simulink model "sailboatModel"  (R2017a)
settings: Solver=ode3  StartTime=0.0  StopTime=200  FixedStep=0.4  RelTol=1e-3
libraries: simulink x2
settings Model: Creator=Administrator  LastModifiedBy=davi
settings DataIOCC: LimitDataPoints=on  SaveFormat=Array  SignalLoggingSaveFormat=ModelDataLogs
settings OptimizationCC: BlockReduction=off  BooleanDataType=off  LifeSpan=inf
settings DebuggingCC: SaveWithParameterizedLinksMsg=none  UnderspecifiedInitializationDetection=Classic  MergeDetectMultiDrivingBlocksExec=none  SignalResolutionControl=TryResolveAllWithWarning  MultiTaskDSMMsg=warning  MultiTaskCondExecSysMsg=none  StateNameClashWarn=warning  SFUnexpectedBacktrackingDiag=warning  SFNoUnconditionalDefaultTransitionDiag=warning  SFExecutionAtInitializationDiag=none
settings HardwareCC: ProdBitPerPointer=32  ProdBitPerSizeT=32  ProdBitPerPtrDiffT=32  ProdLargestAtomicFloat=None  ProdIntDivRoundTo=Undefined  ProdEndianess=Unspecified  ProdWordSize=32  ProdHWDeviceType=32-bit Generic  TargetUnknown=on
settings ModelReferenceCC: PropagateSignalLabelsOutOfModel=off
settings GRTTargetCC: TargetLangStandard=C89/C90 (ANSI)  GeneratePreprocessorConditionals=Disable all
settings ConfigComp: CovMetricSettings=dw  CovHtmlReporting=on  CovSaveCumulativeToWorkspaceVar=on  CovSaveSingleToWorkspaceVar=on  CovExternalEMLEnable=off

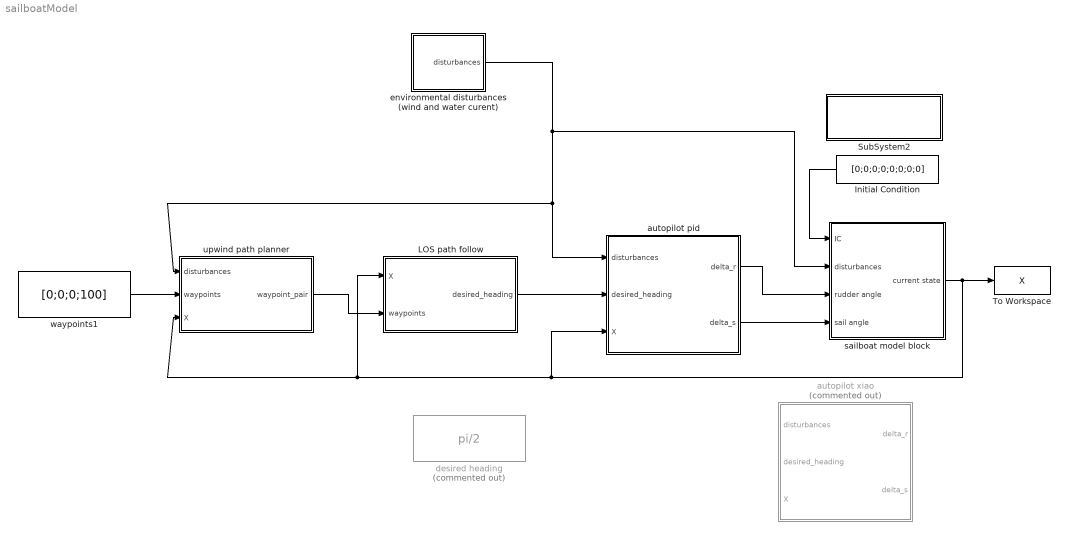
== system sailboatModel ==
  Initial Condition : Constant  Value=[0;0;0;0;0;0;0;0]
  LOS path follow : Subsystem
  SubSystem2 : Subsystem  InitFcn=init_par
      mask Display: disp('Parameter Initialization')
  To Workspace : ToWorkspace  VariableName=X  SaveFormat=Structure With Time  SampleTime=-1
  autopilot pid : Subsystem
  autopilot xiao : Subsystem  Commented=on
  desired heading : Constant  Commented=on  Value=pi/2
  environmental disturbances (wind and water curent) : Subsystem
  sailboat model block : Subsystem  StopFcn=|
      | %close all;
      | %plot(X.signals.values(:,1), X.signals.values(:,2),'r', 'LineWidth', 1.5);
      | %axis([-max(max(X.signals.values(:,1),max(X.signals.values(:,2))))/2 max(max(X.signals.values(:,1),max(X.signals.values(:,2))))/2 min(min(X.signals.values(:,1),min(X.signals.values(:,2)))) max(max(X.signals.values(:,1),max(X.signals.values(:,2))))]);
      | %grid;
      | %xlabel('x[m]');
      | %ylabel('y[m]');
      | %
      | %figure;
      | %hold on;
      | %plot(X.time, rad2deg(X.signals.values(:,4)),'r', 'LineWidth', 1.5);
      | %xlabel('Time[s]');
      | %ylabel('Heading[deg]');
      | %grid;
  upwind path planner : Subsystem
  waypoints1 : Constant  Value=[0;0;0;100]
  wires:
  sailboat model block/1(current state) -> autopilot pid/3(X), LOS path follow/1(X), upwind path planner/3(X), To Workspace/1
  Initial Condition/1 -> sailboat model block/1(IC)
  autopilot pid/1(delta_r) -> sailboat model block/3(rudder angle)
  autopilot pid/2(delta_s) -> sailboat model block/4(sail angle)
  environmental disturbances (wind and water curent)/1(disturbances) -> autopilot pid/1(disturbances), upwind path planner/1(disturbances), sailboat model block/2(disturbances)
  LOS path follow/1(desired_heading) -> autopilot pid/2(desired_heading)
  waypoints1/1 -> upwind path planner/2(waypoints)
  upwind path planner/1(waypoint_pair) -> LOS path follow/2(waypoints)

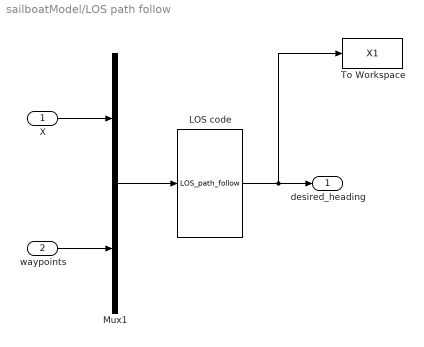
== system sailboatModel/LOS path follow ==
  X : Inport
  waypoints : Inport  Port=2
  LOS code : MATLABFcn  MATLABFcn=LOS_path_follow  OutputDimensions=1
  Mux1 : Mux  Inputs=2
  To Workspace : ToWorkspace  VariableName=X1  SaveFormat=Structure With Time  SampleTime=-1
  desired_heading : Outport
  wires:
  X/1 -> Mux1/1
  Mux1/1 -> LOS code/1
  LOS code/1 -> To Workspace/1, desired_heading/1
  waypoints/1 -> Mux1/2

== system sailboatModel/SubSystem2 ==

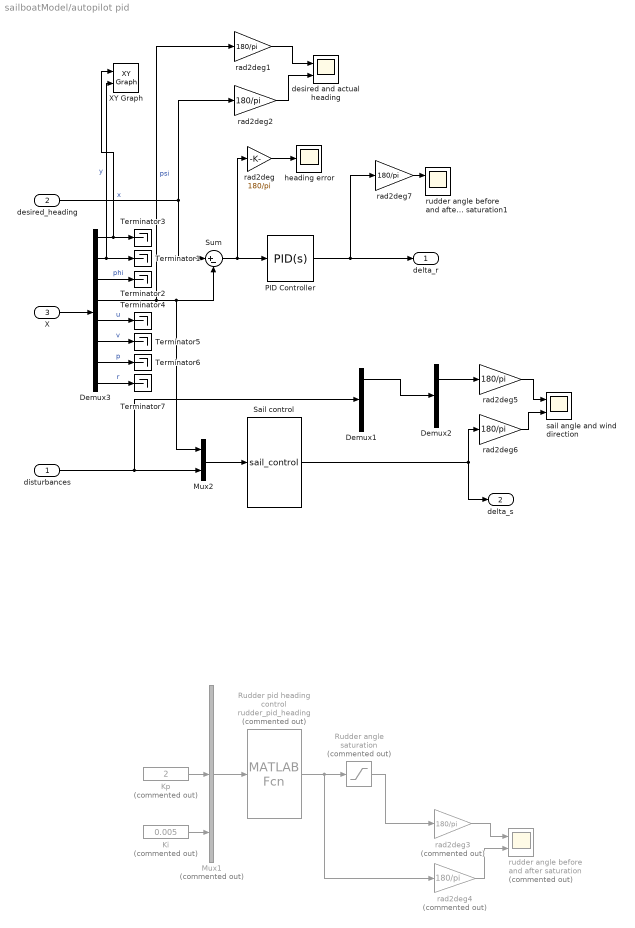
== system sailboatModel/autopilot pid ==
  disturbances : Inport
  desired_heading : Inport  Port=2
  X : Inport  Port=3
  Demux1 : Demux  Outputs=3
  Demux2 : Demux  Outputs=2
  Demux3 : Demux  Outputs=8
  Ki : Constant  Commented=on  Value=0.005
  Kp : Constant  Commented=on  Value=2
  Mux1 : Mux  Commented=on  Inputs=3
  Mux2 : Mux  Inputs=2
  PID Controller : simulink/Continuous/PID Controller  Controller=PID  TimeDomain=Continuous-time  SampleTime=-1  IntegratorMethod=Forward Euler  FilterMethod=Forward Euler  Form=Parallel  UseFilter=on  ControllerParametersSource=internal  P=3  I=0.05  D=0.5  N=1  InitialConditionSource=internal  InitialConditionForIntegrator=0  InitialConditionForFilter=0  ExternalReset=none  LimitOutput=on  UpperSaturationLimit=pi/3  LowerSaturationLimit=-pi/3  LinearizeAsGain=on  AntiWindupMode=clamping  Kb=1  TrackingMode=off  Kt=1  PParamMin=[]  PParamMax=[]  IParamMin=[]  IParamMax=[]  DParamMin=[]  DParamMax=[]  NParamMin=[]  NParamMax=[]  KbParamMin=[]  KbParamMax=[]  KtParamMin=[]  KtParamMax=[]  POutMin=[]  POutMax=[]  IOutMin=[]  IOutMax=[]  DOutMin=[]  DOutMax=[]  NOutMin=[]  NOutMax=[]  KbOutMin=[]  KbOutMax=[]  KtOutMin=[]  KtOutMax=[]  IntegratorOutMin=[]  IntegratorOutMax=[]  FilterOutMin=[]  FilterOutMax=[]  SumOutMin=[]  SumOutMax=[]  SumI1OutMin=[]  SumI1OutMax=[]  SumI2OutMin=[]  SumI2OutMax=[]  SumI3OutMin=[]  SumI3OutMax=[]  SumDOutMin=[]  SumDOutMax=[]  SaturationOutMin=[]  SaturationOutMax=[]  IntegratorContinuousStateAttributes=''  IntegratorStateMustResolveToSignalObject=off  IntegratorRTWStateStorageClass=Auto  FilterContinuousStateAttributes=''  FilterStateMustResolveToSignalObject=off  FilterRTWStateStorageClass=Auto  DifferentiatorICPrevScaledInput=0  DifferentiatorOutMin=[]  DifferentiatorOutMax=[]  InitialConditionSetting=State (most efficient)
  Rudder angle saturation : Saturate  Commented=on  UpperLimit=pi/3  LowerLimit=-pi/3  LinearizeAsGain=off
  Rudder pid heading control : MATLABFcn  Commented=on  MATLABFcn=rudder_pid_heading  OutputDimensions=1
  Sail control : MATLABFcn  MATLABFcn=sail_control  OutputDimensions=1
  Sum : Sum  Inputs=|+-  SaturateOnIntegerOverflow=on
  Terminator{1..7} (7 alike) : Terminator
  XY Graph : simulink/Sinks/XY Graph  xmin=-50  xmax=50  ymin=0  ymax=200  st=-1
  desired and actual heading : Scope  NumInputPorts=2
  heading error : Scope
  rad2deg{,1..2,5..7} (6 alike) : Gain  Gain=180/pi
  rad2deg3 : Gain  Commented=on  Gain=180/pi
  rad2deg4 : Gain  Commented=on  Gain=180/pi
  rudder angle before and after saturation : Scope  Commented=on  NumInputPorts=2
  rudder angle before and after saturation1 : Scope  NumInputPorts=2
  sail angle and wind direction : Scope  NumInputPorts=2
  delta_r : Outport
  delta_s : Outport  Port=2
  wires:
  Demux3/4 -> rad2deg1/1, Mux2/1, Sum/2  "psi"
  X/1 -> Demux3/1
  Demux3/1 -> XY Graph/1, Terminator3/1  "x"
  Demux3/2 -> Terminator1/1, XY Graph/2  "y"
  Demux3/3 -> Terminator2/1  "phi"
  Demux3/5 -> Terminator4/1  "u"
  Demux3/6 -> Terminator5/1  "v"
  Demux3/7 -> Terminator6/1  "p"
  Demux3/8 -> Terminator7/1  "r"
  Rudder angle saturation/1 -> rad2deg3/1
  Rudder pid heading control/1 -> rad2deg4/1, Rudder angle saturation/1
  desired_heading/1 -> Sum/1, rad2deg2/1
  Mux1/1 -> Rudder pid heading control/1
  Sum/1 -> rad2deg/1, PID Controller/1
  Kp/1 -> Mux1/2
  Ki/1 -> Mux1/3
  Sail control/1 -> rad2deg6/1, delta_s/1
  disturbances/1 -> Demux1/1, Mux2/2
  Mux2/1 -> Sail control/1
  rad2deg/1 -> heading error/1
  rad2deg1/1 -> desired and actual heading/1
  rad2deg2/1 -> desired and actual heading/2
  rad2deg3/1 -> rudder angle before and after saturation/1
  rad2deg4/1 -> rudder angle before and after saturation/2
  rad2deg5/1 -> sail angle and wind direction/1
  Demux1/1 -> Demux2/1
  Demux2/1 -> rad2deg5/1
  rad2deg6/1 -> sail angle and wind direction/2
  PID Controller/1 -> rad2deg7/1, delta_r/1
  rad2deg7/1 -> rudder angle before and after saturation1/1

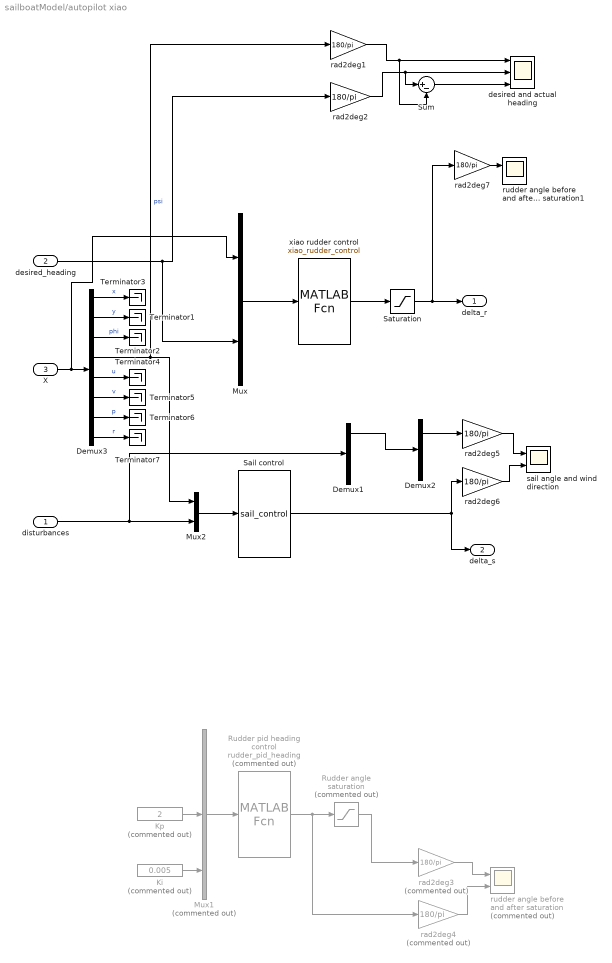
== system sailboatModel/autopilot xiao ==
  disturbances : Inport
  desired_heading : Inport  Port=2
  X : Inport  Port=3
  Demux1 : Demux  Outputs=3
  Demux2 : Demux  Outputs=2
  Demux3 : Demux  Outputs=8
  Ki : Constant  Commented=on  Value=0.005
  Kp : Constant  Commented=on  Value=2
  Mux : Mux  Inputs=2
  Mux1 : Mux  Commented=on  Inputs=3
  Mux2 : Mux  Inputs=2
  Rudder angle saturation : Saturate  Commented=on  UpperLimit=pi/3  LowerLimit=-pi/3  LinearizeAsGain=off
  Rudder pid heading control : MATLABFcn  Commented=on  MATLABFcn=rudder_pid_heading  OutputDimensions=1
  Sail control : MATLABFcn  MATLABFcn=sail_control  OutputDimensions=1
  Saturation : Saturate  UpperLimit=pi/3  LowerLimit=-pi/3
  Sum : Sum  Inputs=|+-  SaturateOnIntegerOverflow=on
  Terminator{1..7} (7 alike) : Terminator
  desired and actual heading : Scope  NumInputPorts=3
  rad2deg{1..2,5..7} (5 alike) : Gain  Gain=180/pi
  rad2deg3 : Gain  Commented=on  Gain=180/pi
  rad2deg4 : Gain  Commented=on  Gain=180/pi
  rudder angle before and after saturation : Scope  Commented=on  NumInputPorts=2
  rudder angle before and after saturation1 : Scope  NumInputPorts=2
  sail angle and wind direction : Scope  NumInputPorts=2
  xiao rudder control : MATLABFcn  MATLABFcn=xiao_rudder_control  OutputDimensions=1
  delta_r : Outport
  delta_s : Outport  Port=2
  wires:
  Demux3/4 -> rad2deg1/1, Mux2/1  "psi"
  X/1 -> Mux/1, Demux3/1
  Demux3/1 -> Terminator3/1  "x"
  Demux3/2 -> Terminator1/1  "y"
  Demux3/3 -> Terminator2/1  "phi"
  Demux3/5 -> Terminator4/1  "u"
  Demux3/6 -> Terminator5/1  "v"
  Demux3/7 -> Terminator6/1  "p"
  Demux3/8 -> Terminator7/1  "r"
  Rudder angle saturation/1 -> rad2deg3/1
  Rudder pid heading control/1 -> rad2deg4/1, Rudder angle saturation/1
  desired_heading/1 -> Mux/2, rad2deg2/1
  Mux1/1 -> Rudder pid heading control/1
  Kp/1 -> Mux1/2
  Ki/1 -> Mux1/3
  Sail control/1 -> rad2deg6/1, delta_s/1
  disturbances/1 -> Demux1/1, Mux2/2
  Mux2/1 -> Sail control/1
  rad2deg1/1 -> Sum/2, desired and actual heading/1
  rad2deg2/1 -> Sum/1, desired and actual heading/2
  rad2deg3/1 -> rudder angle before and after saturation/1
  rad2deg4/1 -> rudder angle before and after saturation/2
  rad2deg5/1 -> sail angle and wind direction/1
  Demux1/1 -> Demux2/1
  Demux2/1 -> rad2deg5/1
  rad2deg6/1 -> sail angle and wind direction/2
  rad2deg7/1 -> rudder angle before and after saturation1/1
  Mux/1 -> xiao rudder control/1
  xiao rudder control/1 -> Saturation/1
  Saturation/1 -> rad2deg7/1, delta_r/1
  Sum/1 -> desired and actual heading/3

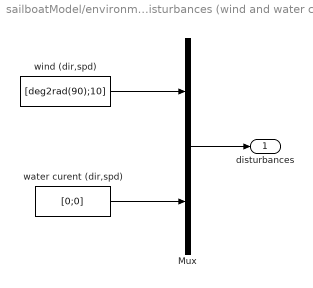
== system sailboatModel/environmental disturbances (wind and water curent) ==
  Mux : Mux  Inputs=2
  water curent (dir,spd) : Constant  Value=[0;0]
  wind (dir,spd) : Constant  Value=[deg2rad(90);10]
  disturbances : Outport
  wires:
  water curent (dir,spd)/1 -> Mux/2
  wind (dir,spd)/1 -> Mux/1
  Mux/1 -> disturbances/1

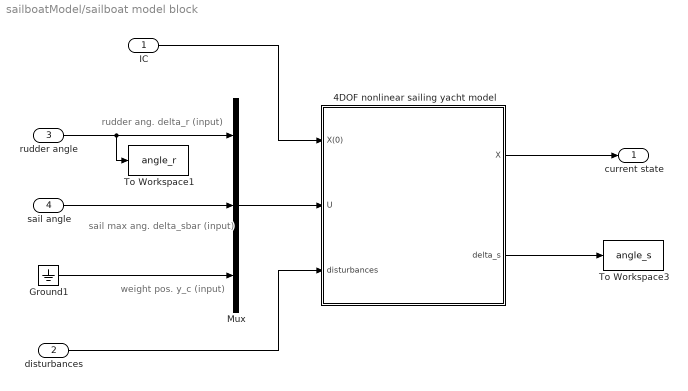
== system sailboatModel/sailboat model block ==
  note: weight pos. y_c (input)
  note: rudder ang. delta_r (input)
  note: sail max ang. delta_sbar (input)
  IC : Inport
  disturbances : Inport  Port=2
  rudder angle : Inport  Port=3
  sail angle : Inport  Port=4
  4DOF nonlinear sailing yacht model : Subsystem
  Ground1 : Ground
  Mux : Mux  Inputs=3
  To Workspace1 : ToWorkspace  VariableName=angle_r  SaveFormat=Structure With Time  SampleTime=-1
  To Workspace3 : ToWorkspace  VariableName=angle_s  SaveFormat=Structure With Time  SampleTime=-1
  current state : Outport
  wires:
  Mux/1 -> 4DOF nonlinear sailing yacht model/2(U)
  4DOF nonlinear sailing yacht model/2(delta_s) -> To Workspace3/1
  sail angle/1 -> Mux/2
  rudder angle/1 -> To Workspace1/1, Mux/1
  4DOF nonlinear sailing yacht model/1(X) -> current state/1
  Ground1/1 -> Mux/3
  IC/1 -> 4DOF nonlinear sailing yacht model/1(X(0))
  disturbances/1 -> 4DOF nonlinear sailing yacht model/3(disturbances)

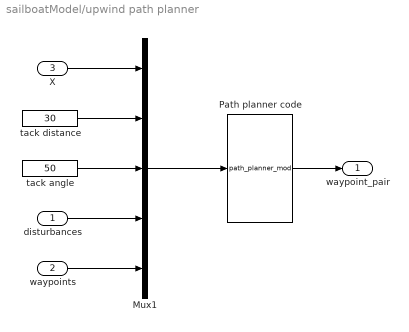
== system sailboatModel/upwind path planner ==
  disturbances : Inport
  waypoints : Inport  Port=2
  X : Inport  Port=3
  Mux1 : Mux  Inputs=5
  Path planner code : MATLABFcn  MATLABFcn=path_planner_mod  OutputDimensions=1
  tack angle : Constant  Value=50
  tack distance : Constant  Value=30
  waypoint_pair : Outport
  wires:
  X/1 -> Mux1/1
  tack distance/1 -> Mux1/2
  tack angle/1 -> Mux1/3
  Mux1/1 -> Path planner code/1
  Path planner code/1 -> waypoint_pair/1
  disturbances/1 -> Mux1/4
  waypoints/1 -> Mux1/5

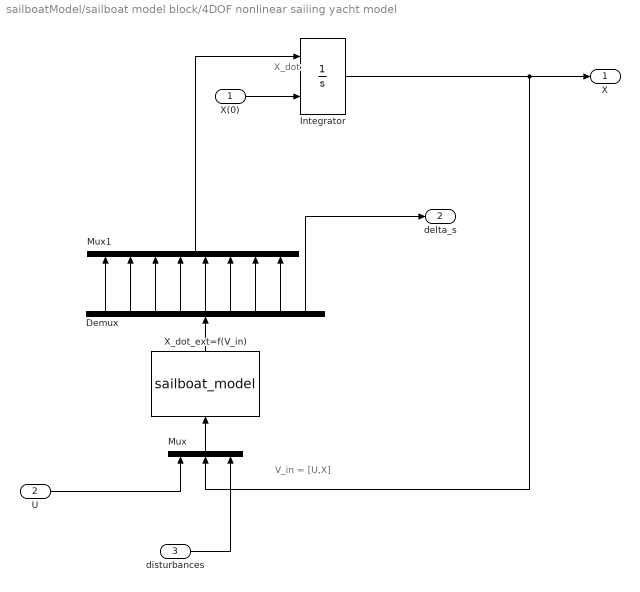
== system sailboatModel/sailboat model block/4DOF nonlinear sailing yacht model ==
  note: X_dot
  note: V_in = [U,X]
  X(0) : Inport
  U : Inport  Port=2
  disturbances : Inport  Port=3
  Demux : Demux  Outputs=9
  Integrator : Integrator  InitialConditionSource=external  InitialCondition=[0;0;0;pi;1;0;0;0]
  Mux : Mux  Inputs=3
  Mux1 : Mux  Inputs=8
  X_dot_ext=f(V_in) : MATLABFcn  MATLABFcn=sailboat_model  OutputDimensions=9
  X : Outport
  delta_s : Outport  Port=2
  wires:
  X(0)/1 -> Integrator/2
  Mux/1 -> X_dot_ext=f(V_in)/1
  U/1 -> Mux/1
  Integrator/1 -> X/1, Mux/2
  X_dot_ext=f(V_in)/1 -> Demux/1
  Demux/9 -> delta_s/1
  Demux/8 -> Mux1/8
  Demux/7 -> Mux1/7
  Demux/6 -> Mux1/6
  Demux/5 -> Mux1/5
  Demux/4 -> Mux1/4
  Demux/3 -> Mux1/3
  Demux/2 -> Mux1/2
  Demux/1 -> Mux1/1
  Mux1/1 -> Integrator/1
  disturbances/1 -> Mux/3
